simulink library "DC_Loads_Lib"  (R2014a)
settings: Solver=ode45  StartTime=0.0  StopTime=10.0  RelTol=1e-3
undefined symbols (not defined in the file): APN_Param, D1, Delta, Hydride, Metal, Nickel, Ts
libraries: powerlib x30, fl_lib x26, nesl_utility x14, DC_Loads_Lib x3, elec_lib x2, electricdrivelib x1, simulink x1, APN_Battery_Lib x1, sh_lib x1
Description:
  | Copyright 2014 The MathWorks, Inc.
settings Model: Creator=smiller  LastModifiedBy=psanghvi

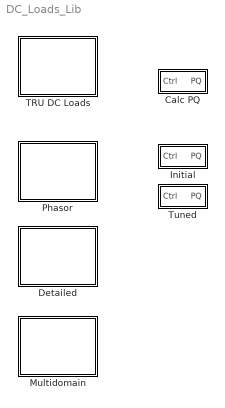
== system DC_Loads_Lib ==
  Calc PQ : Subsystem  BlockChoice=Initial
      settings: TemplateBlock=self  MemberBlocks=Initial,Tuned
  Detailed : Subsystem
      mask Display: image(imread('TRU_Detailed_IMAGE.jpg'));
  Initial : Subsystem
  Multidomain : Subsystem
      mask Display: image(imread('TRU_Multidomain_IMAGE.jpg'));
  Phasor : Subsystem
      mask Display: image(imread('TRU_Phasor_IMAGE.jpg'));
  TRU DC Loads : Subsystem  BlockChoice=Detailed
      settings: TemplateBlock=self  MemberBlocks=Detailed,Multidomain,Phasor
  Tuned : Subsystem

== system DC_Loads_Lib/Calc PQ ==
  Ctrl : Inport
  Initial : DC_Loads_Lib/Initial
  PQ : Outport
  wires:
  Ctrl/1 -> Initial/1
  Initial/1 -> PQ/1

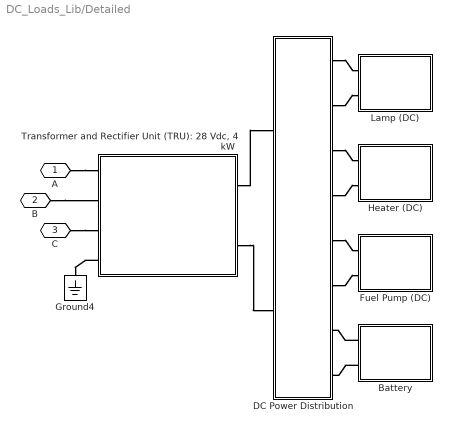
== system DC_Loads_Lib/Detailed ==
  Battery : Subsystem
      mask Display:
      | image(imread('BatteryDC_PS_IMAGE.jpg','jpg'))
      | port_label('LConn',1,'+');
      | port_label('LConn',2,'-');
  "DC Power Distribution " : Subsystem
  Fuel Pump (DC) : Subsystem
      mask Display:
      | image(imread('PumpDC_PS_IMAGE.jpg','jpg'))
      | port_label('LConn',1,'+');
      | port_label('LConn',2,'-');
  Ground4 : powerlib/Elements/Ground  LConnTagsString=a
  Heater (DC) : Subsystem
      mask Display:
      | image(imread('HeaterDC_PS_IMAGE.jpg','jpg'))
      | port_label('LConn',1,'+');
      | port_label('LConn',2,'-');
  Lamp (DC) : Subsystem
      mask Display:
      | image(imread('LampDC_PS_IMAGE.jpg','jpg'))
      | port_label('LConn',1,'+');
      | port_label('LConn',2,'-');
  "Transformer and Rectifier Unit (TRU): 28 Vdc, 4 kW" : Subsystem
      mask Display:
      | image(imread('TRU_PS_IMAGE.jpg','jpg'));
      | port_label('LConn',1,'A');
      | port_label('LConn',2,'B');
      | port_label('LConn',3,'C');
      | port_label('LConn',4,'N');
      | port_label('RConn',1,'+');
      | port_label('RConn',2,'-');
  A : PMIOPort  Port=1  Side=Left
  B : PMIOPort  Port=2  Side=Left
  C : PMIOPort  Port=3  Side=Left
  connections:
  A/RConn1 -- "Transformer and Rectifier Unit (TRU): 28 Vdc, 4 kW"/LConn1
  C/RConn1 -- "Transformer and Rectifier Unit (TRU): 28 Vdc, 4 kW"/LConn3
  B/RConn1 -- "Transformer and Rectifier Unit (TRU): 28 Vdc, 4 kW"/LConn2
  "Transformer and Rectifier Unit (TRU): 28 Vdc, 4 kW"/RConn2 -- "DC Power Distribution "/LConn2
  "DC Power Distribution "/RConn6 -- Fuel Pump (DC)/LConn2
  "DC Power Distribution "/RConn1 -- Lamp (DC)/LConn1
  "DC Power Distribution "/RConn5 -- Fuel Pump (DC)/LConn1
  "DC Power Distribution "/RConn2 -- Lamp (DC)/LConn2
  "Transformer and Rectifier Unit (TRU): 28 Vdc, 4 kW"/RConn1 -- "DC Power Distribution "/LConn1
  "Transformer and Rectifier Unit (TRU): 28 Vdc, 4 kW"/LConn4 -- Ground4/LConn1
  "DC Power Distribution "/RConn3 -- Heater (DC)/LConn1
  "DC Power Distribution "/RConn4 -- Heater (DC)/LConn2
  Battery/LConn1 -- "DC Power Distribution "/RConn7
  Battery/LConn2 -- "DC Power Distribution "/RConn8

== system DC_Loads_Lib/Initial ==
  Ctrl : Inport
  Bus Selector1 : BusSelector  OutputSignals=TRU_B
  Constant : Constant  Value=APN_Param.TRU.P
  Constant1 : Constant  Value=APN_Param.TRU.Q
  Filter : Subsystem  mask(First-order lag supporting vector signals){b=1e-2, x_initial=[APN_Param.TRU.P APN_Param.TRU.Q]*0}
      mask prompts: b "Filter time constant"; x_initial "Initial output"
      mask help: Models a lag of the form 1/(b*s+1) where s is the Laplace operator.
  Mux : Mux  Inputs=2
  Product : Product
  PQ : Outport
  wires:
  Product/1 -> Filter/1(In)
  Filter/1(Out) -> PQ/1
  Bus Selector1/1 -> Product/2  "<TRU_B>"
  Mux/1 -> Product/1
  Ctrl/1 -> Bus Selector1/1
  Constant/1 -> Mux/1
  Constant1/1 -> Mux/2

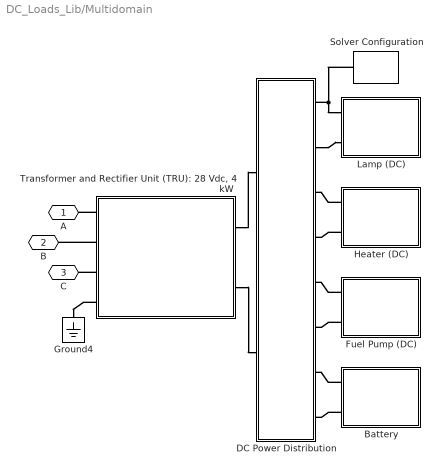
== system DC_Loads_Lib/Multidomain ==
  Battery : Subsystem
      mask Display:
      | image(imread('BatteryDC_SS_IMAGE.jpg','jpg'))
      | port_label('LConn',1,'+');
      | port_label('LConn',2,'-');
  "DC Power Distribution " : Subsystem
  Fuel Pump (DC) : Subsystem
      mask Display:
      | image(imread('PumpDC_SS_IMAGE.jpg','jpg'))
      | port_label('LConn',1,'+');
      | port_label('LConn',2,'-');
  Ground4 : powerlib/Elements/Ground  LConnTagsString=a
  Heater (DC) : Subsystem
      mask Display:
      | image(imread('HeaterDC_SS_IMAGE.jpg','jpg'))
      | port_label('LConn',1,'+');
      | port_label('LConn',2,'-');
  Lamp (DC) : Subsystem
      mask Display:
      | image(imread('LampDC_SS_IMAGE.jpg','jpg'))
      | port_label('LConn',1,'+');
      | port_label('LConn',2,'-');
  Solver Configuration : nesl_utility/Solver Configuration  PhysicalDomain=network_engine_domain  SubClassName=solver  LeftPortType=input  RightPortType=generic  Accelerate=off  Tones=[]  Harmonics=[]  SimulateNoise=off  Profile=off  UseLocalSampling=off  EnableSwitchedLinearOptims=on  FrequencyDomain=off  UseCCode=off  RelTol=0.001  AbsTol=1e-06  MinStep=1e-09  ToWorkspace=off  DoDC=off  ResidualTolerance=1e-9  UseLocalSolver=on  LocalSolverChoice=NE_BACKWARD_EULER_ADVANCER  LocalSolverSampleTime=Ts  DoFixedCost=on  MaxNonlinIter=3  MaxModeIter=2  LinearAlgebra=Sparse  DelaysMemoryBudget=1024  AutomaticFiltering=on  FilteringTimeConstant=0.001
  "Transformer and Rectifier Unit (TRU): 28 Vdc, 4 kW" : Subsystem
      mask Display:
      | image(imread('TRU_PSSS_IMAGE.jpg','jpg'));
      | port_label('LConn',1,'A');
      | port_label('LConn',2,'B');
      | port_label('LConn',3,'C');
      | port_label('LConn',4,'N');
      | port_label('RConn',1,'+');
      | port_label('RConn',2,'-');
  A : PMIOPort  Port=1  Side=Left
  B : PMIOPort  Port=2  Side=Left
  C : PMIOPort  Port=3  Side=Left
  connections:
  Battery/LConn2 -- "DC Power Distribution "/RConn8
  Battery/LConn1 -- "DC Power Distribution "/RConn7
  "Transformer and Rectifier Unit (TRU): 28 Vdc, 4 kW"/RConn2 -- "DC Power Distribution "/LConn2
  "Transformer and Rectifier Unit (TRU): 28 Vdc, 4 kW"/RConn1 -- "DC Power Distribution "/LConn1
  Fuel Pump (DC)/LConn1 -- "DC Power Distribution "/RConn5
  Fuel Pump (DC)/LConn2 -- "DC Power Distribution "/RConn6
  Heater (DC)/LConn1 -- "DC Power Distribution "/RConn3
  Heater (DC)/LConn2 -- "DC Power Distribution "/RConn4
  "DC Power Distribution "/RConn1 -- Lamp (DC)/LConn1 -- Solver Configuration/RConn1
  "DC Power Distribution "/RConn2 -- Lamp (DC)/LConn2
  "Transformer and Rectifier Unit (TRU): 28 Vdc, 4 kW"/LConn1 -- A/RConn1
  "Transformer and Rectifier Unit (TRU): 28 Vdc, 4 kW"/LConn3 -- C/RConn1
  "Transformer and Rectifier Unit (TRU): 28 Vdc, 4 kW"/LConn2 -- B/RConn1
  "Transformer and Rectifier Unit (TRU): 28 Vdc, 4 kW"/LConn4 -- Ground4/LConn1

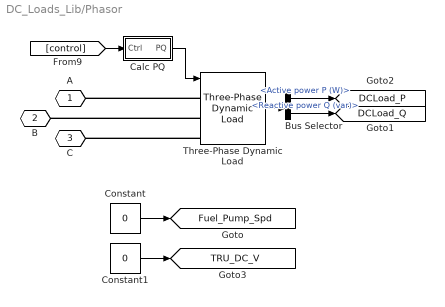
== system DC_Loads_Lib/Phasor ==
  Bus Selector : BusSelector  OutputSignals=Active power P (W),Reactive power Q (var)
  Calc PQ : Subsystem  BlockChoice=Tuned
      settings: AttributesFormatString=%<BlockChoice>  TemplateBlock=DC_Loads_Lib/Calc PQ  MemberBlocks=Initial,Tuned
  Constant : Constant  Value=0
  Constant1 : Constant  Value=0
  Three-Phase Dynamic Load : powerlib/Elements/Three-Phase Dynamic Load  NominalVoltage=[ 500e3 400 ]  ActiveReactivePowers=[APN_Param.TRU.P APN_Param.TRU.Q]  PositiveSequence=[0.0004 0]  ExternalControl=on  NpNq=[1.3 2]  TimeConstants="[0  0  0  0]"  MinimumVoltage=0.7  LoadFlowParameters=[4 0 0 0 0]
  A : PMIOPort  Port=1  Side=Left
  B : PMIOPort  Port=2  Side=Left
  C : PMIOPort  Port=3  Side=Left
  tag scope: DCLoad_P=global, DCLoad_Q=global, Fuel_Pump_Spd=global, TRU_DC_V=global
  wires:
  Bus Selector/1 -> [DCLoad_P]  "<Active power P (W)>"
  Three-Phase Dynamic Load/1 -> Bus Selector/1
  Constant/1 -> [Fuel_Pump_Spd]
  Bus Selector/2 -> [DCLoad_Q]  "<Reactive power Q (var)>"
  [control] -> Calc PQ/1(Ctrl)
  Calc PQ/1(PQ) -> Three-Phase Dynamic Load/1
  Constant1/1 -> [TRU_DC_V]
  connections:
  Three-Phase Dynamic Load/LConn3 -- C/RConn1
  Three-Phase Dynamic Load/LConn2 -- B/RConn1
  Three-Phase Dynamic Load/LConn1 -- A/RConn1

== system DC_Loads_Lib/TRU DC Loads ==
  Detailed : DC_Loads_Lib/Detailed  SystemSampleTime=-1
  A : PMIOPort  Port=1  Side=Left
  B : PMIOPort  Port=2  Side=Left
  C : PMIOPort  Port=3  Side=Left
  connections:
  Detailed/LConn1 -- A/RConn1
  Detailed/LConn2 -- B/RConn1
  Detailed/LConn3 -- C/RConn1

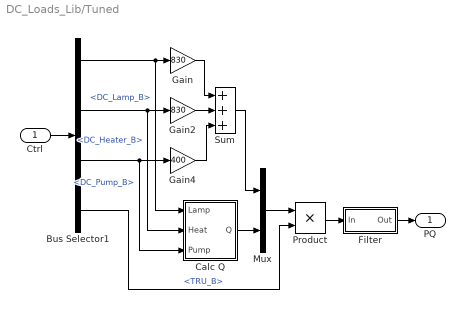
== system DC_Loads_Lib/Tuned ==
  Ctrl : Inport
  Bus Selector1 : BusSelector  OutputSignals=TRU_B_Bus.DC_Lamp_B,TRU_B_Bus.DC_Heater_B,TRU_B_Bus.DC_Pump_B,TRU_B
  Calc Q : Subsystem
  Filter : Subsystem  mask(First-order lag supporting vector signals){b=1e-2, x_initial=0}
      mask prompts: b "Filter time constant"; x_initial "Initial output"
      mask help: Models a lag of the form 1/(b*s+1) where s is the Laplace operator.
  Gain : Gain  Gain=830
  Gain2 : Gain  Gain=830
  Gain4 : Gain  Gain=400
  Mux : Mux  Inputs=2
  Product : Product
  Sum : Sum  Inputs=+++
  PQ : Outport
  wires:
  Ctrl/1 -> Bus Selector1/1
  Bus Selector1/1 -> Calc Q/1(Lamp), Gain/1  "<DC_Lamp_B>"
  Sum/1 -> Mux/1
  Mux/1 -> Product/1
  Bus Selector1/2 -> Calc Q/2(Heat), Gain2/1  "<DC_Heater_B>"
  Bus Selector1/3 -> Calc Q/3(Pump), Gain4/1  "<DC_Pump_B>"
  Gain/1 -> Sum/1
  Gain2/1 -> Sum/2
  Gain4/1 -> Sum/3
  Bus Selector1/4 -> Product/2  "<TRU_B>"
  Filter/1(Out) -> PQ/1
  Product/1 -> Filter/1(In)
  Calc Q/1(Q) -> Mux/2

== system DC_Loads_Lib/Detailed/Battery ==
  Battery : electricdrivelib/Extra Sources/Battery  BatType=Nickel-Metal-Hydride  ShowDetailedParameters=off  NomV=28  NomQ=12  SOC=100  PresetModel=on  MaxQ=12.9231  FullV=32.9831  Dis_rate=2.4  R=0.023333  Normal_OP=11.5385  expZone="[30.3729          2.4]"  Dis_Char=off  current=[1.5 3]  Units=Ampere-hour  Batt_Tr=30
  Terminator : Terminator
  + : PMIOPort  Port=1  Side=Left
  - : PMIOPort  Port=2  Side=Left
  wires:
  Battery/1 -> Terminator/1
  connections:
  Battery/LConn1 -- +/RConn1
  Battery/LConn2 -- -/RConn1

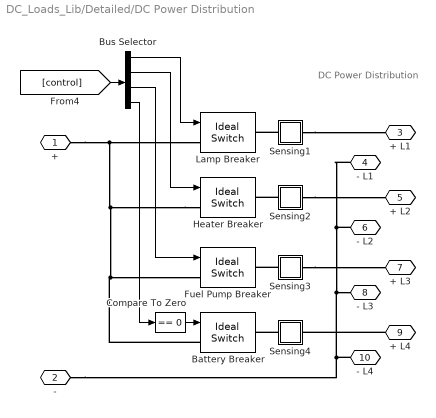
== system DC_Loads_Lib/Detailed/DC Power Distribution  ==
  note: DC Power Distribution
  Battery Breaker : powerlib/Power Electronics/Ideal Switch  Ron=0.001  Lon=0  IC=0  Rs=1e3  Cs=inf  Measurements=off
  Bus Selector : BusSelector  OutputSignals=TRU_B_Bus.DC_Lamp_B,TRU_B_Bus.DC_Heater_B,TRU_B_Bus.DC_Pump_B,TRU_B
  Compare To Zero : simulink/Logic and Bit Operations/Compare To Zero  relop===  OutDataTypeStr=boolean
  Fuel Pump Breaker : powerlib/Power Electronics/Ideal Switch  Ron=0.001  Lon=0  IC=0  Rs=1e3  Cs=inf  Measurements=off
  Heater Breaker : powerlib/Power Electronics/Ideal Switch  Ron=0.001  Lon=0  IC=0  Rs=1e3  Cs=inf  Measurements=off
  Lamp Breaker : powerlib/Power Electronics/Ideal Switch  Ron=0.001  Lon=0  IC=0  Rs=1e3  Cs=inf  Measurements=off
  Sensing1 : Subsystem
      mask Display: disp('S');
  Sensing2 : Subsystem
      mask Display: disp('S');
  Sensing3 : Subsystem
      mask Display: disp('S');
  Sensing4 : Subsystem
      mask Display: disp('S');
  + : PMIOPort  Port=1  Side=Left
  - : PMIOPort  Port=2  Side=Left
  + L1 : PMIOPort  Port=3  Side=Right
  - L1 : PMIOPort  Port=4  Side=Right
  + L2 : PMIOPort  Port=5  Side=Right
  - L2 : PMIOPort  Port=6  Side=Right
  + L3 : PMIOPort  Port=7  Side=Right
  - L3 : PMIOPort  Port=8  Side=Right
  + L4 : PMIOPort  Port=9  Side=Right
  - L4 : PMIOPort  Port=10  Side=Right
  wires:
  Bus Selector/3 -> Fuel Pump Breaker/1
  Bus Selector/2 -> Heater Breaker/1
  Bus Selector/1 -> Lamp Breaker/1
  [control] -> Bus Selector/1
  Bus Selector/4 -> Compare To Zero/1
  Compare To Zero/1 -> Battery Breaker/1
  connections:
  - L2/RConn1 -- - L1/RConn1 -- - L3/RConn1 -- - L4/RConn1 -- -/RConn1
  Heater Breaker/LConn1 -- Battery Breaker/LConn1 -- Fuel Pump Breaker/LConn1 -- Lamp Breaker/LConn1 -- +/RConn1
  Sensing1/LConn1 -- Lamp Breaker/RConn1
  Sensing1/RConn1 -- + L1/RConn1
  Sensing2/LConn1 -- Heater Breaker/RConn1
  Sensing2/RConn1 -- + L2/RConn1
  Sensing3/LConn1 -- Fuel Pump Breaker/RConn1
  Sensing3/RConn1 -- + L3/RConn1
  Sensing4/LConn1 -- Battery Breaker/RConn1
  + L4/RConn1 -- Sensing4/RConn1

== system DC_Loads_Lib/Detailed/Fuel Pump (DC) ==
  Bus Selector : BusSelector  OutputSignals=Speed wm (rad/s)
  DC Machine : powerlib/Machines/DC Machine  PresetModel=No  MechanicalLoad=Torque TL  FieldType=Wound  ShowDetailedParameters=on  MeasurementBus=off  RLa=[ .35 0.0001]  RLf="[ 240  12]"  Laf=1  MachineConstant=Torque constant (N.m/A)  Ke=1.8  Kt=1.8  J=0.0005  Bm=0  Tf=0  w0=0  Ifinit=0  TsPowergui=0  TsBlock=-1
  Gain : Gain  Gain=1.5/200
  + : PMIOPort  Port=1  Side=Left
  - : PMIOPort  Port=2  Side=Left
  tag scope: Fuel_Pump_Spd=global
  wires:
  Bus Selector/1 -> Gain/1, [Fuel_Pump_Spd]  "<Speed wm (rad/s)>"
  DC Machine/1 -> Bus Selector/1
  Gain/1 -> DC Machine/1
  connections:
  DC Machine/LConn2 -- DC Machine/LConn1 -- +/RConn1
  DC Machine/RConn2 -- DC Machine/RConn1 -- -/RConn1

== system DC_Loads_Lib/Detailed/Heater (DC) ==
  note: DC Load
  Series RLC Branch3 : powerlib/Elements/Series RLC Branch  LConnTagsString=__new0  RConnTagsString=__new0  BranchType=R  Resistance=1  Inductance=[]  SetiL0=off  InitialCurrent=0  Capacitance=[]  Setx0=off  InitialVoltage=0  Measurements=Branch voltage and current
  + : PMIOPort  Port=1  Side=Left
  - : PMIOPort  Port=2  Side=Left
  connections:
  +/RConn1 -- Series RLC Branch3/LConn1
  -/RConn1 -- Series RLC Branch3/RConn1

== system DC_Loads_Lib/Detailed/Lamp (DC) ==
  note: DC Load
  Series RLC Branch3 : powerlib/Elements/Series RLC Branch  LConnTagsString=__new0  RConnTagsString=__new0  BranchType=R  Resistance=1  Inductance=[]  SetiL0=off  InitialCurrent=0  Capacitance=[]  Setx0=off  InitialVoltage=0  Measurements=Branch voltage and current
  + : PMIOPort  Port=1  Side=Left
  - : PMIOPort  Port=2  Side=Left
  connections:
  -/RConn1 -- Series RLC Branch3/RConn1
  +/RConn1 -- Series RLC Branch3/LConn1

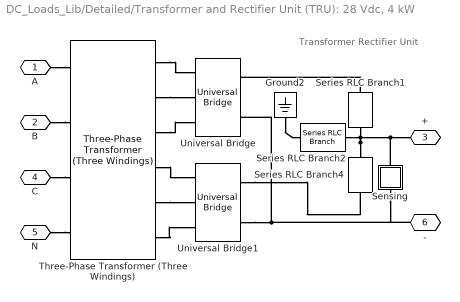
== system DC_Loads_Lib/Detailed/Transformer and Rectifier Unit (TRU): 28 Vdc, 4 kW ==
  note: Transformer Rectifier Unit
  Ground2 : powerlib/Elements/Ground  LConnTagsString=a
  Sensing : Subsystem
  Series RLC Branch1 : powerlib/Elements/Series RLC Branch  LConnTagsString=__new0  RConnTagsString=__new0  BranchType=L  Resistance=[]  Inductance=2e-3  SetiL0=on  InitialCurrent=0  Capacitance=[]  Setx0=off  InitialVoltage=0  Measurements=Branch voltage and current
  Series RLC Branch2 : powerlib/Elements/Series RLC Branch  LConnTagsString=__new0  RConnTagsString=__new0  BranchType=C  Resistance=[]  Inductance=[]  SetiL0=off  InitialCurrent=0  Capacitance=1e-6  Setx0=off  InitialVoltage=0  Measurements=None
  Series RLC Branch4 : powerlib/Elements/Series RLC Branch  LConnTagsString=__new0  RConnTagsString=__new0  BranchType=L  Resistance=[]  Inductance=2e-3  SetiL0=off  InitialCurrent=0  Capacitance=[]  Setx0=off  InitialVoltage=0  Measurements=Branch voltage and current
  Three-Phase Transformer (Three Windings) : powerlib/Elements/Three-Phase Transformer (Three Windings)  Winding1Connection=Yn  UNITS=pu  NominalPower=[ 4200 , 400 ]  Winding1=[ 200 , 0.0002 , 0 ]  Winding2Connection=Delta (D1)  Winding2=[ 22 , 0.0002 , 0 ]  Winding3Connection=Delta (D1)  Winding3=[ 22 , 0.0002 , 0]  SetSaturation=off  Rm=500  Lm=500*10  Saturation=[ 0,0 ; 0.0024,1.2 ; 1.0,1.52 ]  Hysteresis=off  DataFile='hysteresis'  SetInitialFlux=off  InitialFluxes=[0.8 -0.8 0.7]  Measurements=None  MoreParameters=off  BreakLoop=off  DataType=off  TransfoNumber=0
  Universal Bridge : powerlib/Power Electronics/Universal Bridge  Arms=3  SnubberResistance=1e3  SnubberCapacitance=1e-6  Device=Diodes  Ron=1e-3  Lon=0  ForwardVoltages="[  0  0  ]"  ForwardVoltage=0.8  GTOparameters=[ 10e-6 , 20e-6 ]  IGBTparameters=[ 1e-6 , 2e-6 ]  Measurements=None  Measurements_2=None  converterType=Rectifier
  Universal Bridge1 : powerlib/Power Electronics/Universal Bridge  Arms=3  SnubberResistance=1e3  SnubberCapacitance=1e-6  Device=Diodes  Ron=1e-3  Lon=0  ForwardVoltages="[  0  0  ]"  ForwardVoltage=0.8  GTOparameters=[ 10e-6 , 20e-6 ]  IGBTparameters=[ 1e-6 , 2e-6 ]  Measurements=None  Measurements_2=None  converterType=Rectifier
  A : PMIOPort  Port=1  Side=Left
  B : PMIOPort  Port=2  Side=Left
  + : PMIOPort  Port=3  Side=Right
  C : PMIOPort  Port=4  Side=Left
  N : PMIOPort  Port=5  Side=Left
  - : PMIOPort  Port=6  Side=Right
  connections:
  Universal Bridge1/RConn1 -- Series RLC Branch4/RConn1
  Three-Phase Transformer (Three Windings)/RConn6 -- Universal Bridge1/LConn3
  Three-Phase Transformer (Three Windings)/RConn5 -- Universal Bridge1/LConn2
  Three-Phase Transformer (Three Windings)/RConn4 -- Universal Bridge1/LConn1
  Series RLC Branch4/LConn1 -- Sensing/RConn1 -- +/RConn1 -- Series RLC Branch2/LConn1 -- Series RLC Branch1/RConn1
  Series RLC Branch1/LConn1 -- Universal Bridge/RConn1
  N/RConn1 -- Three-Phase Transformer (Three Windings)/LConn4
  C/RConn1 -- Three-Phase Transformer (Three Windings)/LConn3
  B/RConn1 -- Three-Phase Transformer (Three Windings)/LConn2
  A/RConn1 -- Three-Phase Transformer (Three Windings)/LConn1
  Three-Phase Transformer (Three Windings)/RConn3 -- Universal Bridge/LConn3
  Three-Phase Transformer (Three Windings)/RConn2 -- Universal Bridge/LConn2
  Three-Phase Transformer (Three Windings)/RConn1 -- Universal Bridge/LConn1
  Universal Bridge1/RConn2 -- -/RConn1 -- Sensing/LConn1 -- Universal Bridge/RConn2
  Ground2/LConn1 -- Series RLC Branch2/RConn1

== system DC_Loads_Lib/Initial/Filter ==
  In : Inport
  Gain : Gain  Gain=1/b
  Integrator : Integrator  InitialCondition=x_initial
  Sum : Sum  Inputs=|+-  SaturateOnIntegerOverflow=on  InputSameDT=on  OutDataTypeStr=Inherit: Same as first input
  Out : Outport
  wires:
  Gain/1 -> Out/1, Sum/2
  Integrator/1 -> Gain/1
  In/1 -> Sum/1
  Sum/1 -> Integrator/1

== system DC_Loads_Lib/Multidomain/Battery ==
  Ambient temperature : fl_lib/Physical Signals/Sources/PS Constant  constant=273+25
  Battery cell : APN_Battery_Lib/Battery cell  SystemSampleTime=-1
  Convective Heat Transfer : fl_lib/Thermal/Thermal Elements/Convective Heat Transfer  area=Area m^2  heat_tr_coeff=Rtheta W/(m^2 * K)  Q_specify=off  Q_priority=High  Q=0 J/s  T_specify=off  T_priority=High  T=0 K
  Ideal Temperature Source : fl_lib/Thermal/Thermal Sources/Ideal Temperature Source
  Thermal Reference : fl_lib/Thermal/Thermal Elements/Thermal Reference
  + : PMIOPort  Port=1  Side=Left
  - : PMIOPort  Port=2  Side=Left
  connections:
  Battery cell/RConn1 -- -/RConn1
  +/RConn1 -- Battery cell/LConn1
  Thermal Reference/LConn1 -- Ideal Temperature Source/RConn2
  Ideal Temperature Source/RConn1 -- Ambient temperature/RConn1
  Ideal Temperature Source/LConn1 -- Convective Heat Transfer/LConn1
  Convective Heat Transfer/RConn1 -- Battery cell/LConn2

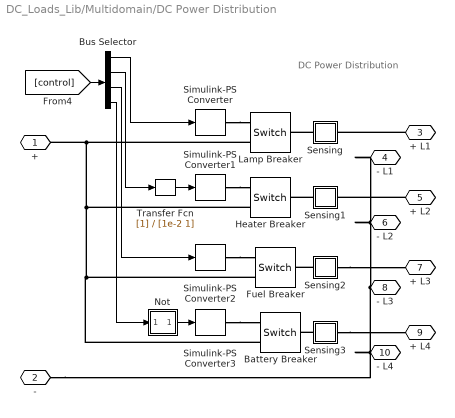
== system DC_Loads_Lib/Multidomain/DC Power Distribution  ==
  note: DC Power Distribution
  Battery Breaker : fl_lib/Electrical/Electrical Elements/Switch  R_closed=0.001 Ohm  G_open=1e-8 1/Ohm  Threshold=0  i_specify=off  i_priority=High  i=0 A  v_specify=off  v_priority=High  v=0 V
  Bus Selector : BusSelector  OutputSignals=TRU_B_Bus.DC_Lamp_B,TRU_B_Bus.DC_Heater_B,TRU_B_Bus.DC_Pump_B,TRU_B
  Fuel Breaker : fl_lib/Electrical/Electrical Elements/Switch  R_closed=0.001 Ohm  G_open=1e-8 1/Ohm  Threshold=0  i_specify=off  i_priority=High  i=0 A  v_specify=off  v_priority=High  v=0 V
  Heater Breaker : fl_lib/Electrical/Electrical Elements/Switch  R_closed=0.001 Ohm  G_open=1e-8 1/Ohm  Threshold=0  i_specify=off  i_priority=High  i=0 A  v_specify=off  v_priority=High  v=0 V
  Lamp Breaker : fl_lib/Electrical/Electrical Elements/Switch  R_closed=0.001 Ohm  G_open=1e-8 1/Ohm  Threshold=0  i_specify=off  i_priority=High  i=0 A  v_specify=off  v_priority=High  v=0 V
  Not : Subsystem
      mask Display: disp('Not')
  Sensing : Subsystem
      mask Display: disp('S');
  Sensing1 : Subsystem
      mask Display: disp('S');
  Sensing2 : Subsystem
      mask Display: disp('S');
  Sensing3 : Subsystem
      mask Display: disp('S');
  Simulink-PS Converter{,1..3} (4 alike) : nesl_utility/Simulink-PS Converter  PhysicalDomain=network_engine_domain  SubClassName=ps_input  LeftPortType=input  RightPortType=output  PseudoPeriodic=off  Frequencies=[]  NoiseDistribution=none  NoiseParameters=[]  Unit=1  AffineConversion=off  InputFiltering=off  SimscapeFilterOrder=1  InputFilterTimeConstant=0.001  UdotUserProvided=1
  Transfer Fcn : TransferFcn  Denominator=[1e-2 1]
  + : PMIOPort  Port=1  Side=Left
  - : PMIOPort  Port=2  Side=Left
  + L1 : PMIOPort  Port=3  Side=Right
  - L1 : PMIOPort  Port=4  Side=Right
  + L2 : PMIOPort  Port=5  Side=Right
  - L2 : PMIOPort  Port=6  Side=Right
  + L3 : PMIOPort  Port=7  Side=Right
  - L3 : PMIOPort  Port=8  Side=Right
  + L4 : PMIOPort  Port=9  Side=Right
  - L4 : PMIOPort  Port=10  Side=Right
  wires:
  Transfer Fcn/1 -> Simulink-PS Converter1/1
  Not/1(Out1) -> Simulink-PS Converter3/1
  Bus Selector/4 -> Not/1(In1)
  [control] -> Bus Selector/1
  Bus Selector/1 -> Simulink-PS Converter/1
  Bus Selector/2 -> Transfer Fcn/1
  Bus Selector/3 -> Simulink-PS Converter2/1
  connections:
  Sensing3/LConn1 -- Battery Breaker/LConn1
  Sensing2/LConn1 -- Fuel Breaker/LConn1
  Simulink-PS Converter3/RConn1 -- Battery Breaker/RConn1
  Simulink-PS Converter2/RConn1 -- Fuel Breaker/RConn1
  Sensing1/LConn1 -- Heater Breaker/LConn1
  Simulink-PS Converter1/RConn1 -- Heater Breaker/RConn1
  + L1/RConn1 -- Sensing/RConn1
  +/RConn1 -- Heater Breaker/RConn2 -- Fuel Breaker/RConn2 -- Battery Breaker/RConn2 -- Lamp Breaker/RConn2
  Sensing/LConn1 -- Lamp Breaker/LConn1
  Simulink-PS Converter/RConn1 -- Lamp Breaker/RConn1
  Sensing3/RConn1 -- + L4/RConn1
  -/RConn1 -- - L4/RConn1 -- - L3/RConn1 -- - L1/RConn1 -- - L2/RConn1
  + L2/RConn1 -- Sensing1/RConn1
  Sensing2/RConn1 -- + L3/RConn1

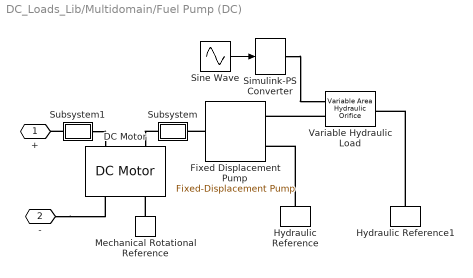
== system DC_Loads_Lib/Multidomain/Fuel Pump (DC) ==
  DC Motor : elec_lib/Actuators & Drivers/Rotational Actuators/DC Motor  parameterization=1  Ra=0.35 Ohm  La=1e-4 H  emf_or_torque=1  Kv=7.2e-5 V/rpm  Ki=6.876e-4 N*m/A  T_stall=2.4e-4 N*m  w_max=1.91e+4 rpm  w_rated=1.5e+4 rpm  P_rated=0.08 W  V_rated=1.5 V  J=5e-4 kg*m^2  lam_param=1  lam=1.5/200 N*m/(rad/s)  i_noload=0 A  V_i_noload=1.5 V  speed0=0 rpm  alpha=0.00393 1/K  Tmeas=25 C  thermal_mass=100 J/K  initial_temperature=25 C
  Fixed Displacement Pump : sh_lib/Pumps and Motors/Fixed-Displacement Pump  D=5e-6 m^3/rad  efficiency_vol=0.92  efficiency_tot=0.8  pr_nominal=1e+7 Pa  w_nominal=188 rad/s  visc_nominal=18 cSt  dens_nominal=900 kg/m^3  k_leak=1e-11 m^3/s/Pa  efficiency_mech=0.7
  Hydraulic Reference : fl_lib/Hydraulic/Hydraulic Elements/Hydraulic Reference
  Hydraulic Reference1 : fl_lib/Hydraulic/Hydraulic Elements/Hydraulic Reference
  Mechanical Rotational Reference : fl_lib/Mechanical/Rotational Elements/Mechanical Rotational Reference
  Simulink-PS Converter : nesl_utility/Simulink-PS Converter  PhysicalDomain=network_engine_domain  SubClassName=ps_input  LeftPortType=input  RightPortType=output  PseudoPeriodic=off  Frequencies=[]  NoiseDistribution=none  NoiseParameters=[]  Unit=1  AffineConversion=off  InputFiltering=on  SimscapeFilterOrder=1  InputFilterTimeConstant=.001  UdotUserProvided=1
  Sine Wave : Sin  Amplitude=1e-4  Bias=1e-3  Frequency=2  SampleTime=0
  Subsystem : Subsystem
      mask Display: disp('S')
  Subsystem1 : Subsystem
      mask Display: disp('S')
  Variable Hydraulic Load : fl_lib/Hydraulic/Hydraulic Elements/Variable Area Hydraulic Orifice  C_d=0.7  Re_cr=12  min_area=1e-12 m^2  q_specify=off  q_priority=High  q=1 m^3/s  p_specify=off  p_priority=High  p=0 Pa
  + : PMIOPort  Port=1  Side=Left
  - : PMIOPort  Port=2  Side=Left
  wires:
  Sine Wave/1 -> Simulink-PS Converter/1
  connections:
  Simulink-PS Converter/RConn1 -- Variable Hydraulic Load/LConn1
  Hydraulic Reference1/LConn1 -- Variable Hydraulic Load/RConn1
  Variable Hydraulic Load/LConn2 -- Fixed Displacement Pump/RConn1
  Hydraulic Reference/LConn1 -- Fixed Displacement Pump/RConn2
  Fixed Displacement Pump/LConn1 -- Subsystem/RConn1
  Subsystem1/RConn1 -- DC Motor/LConn1
  Subsystem1/LConn1 -- +/RConn1
  Subsystem/LConn1 -- DC Motor/LConn2
  Mechanical Rotational Reference/LConn1 -- DC Motor/RConn2
  -/RConn1 -- DC Motor/RConn1

== system DC_Loads_Lib/Multidomain/Heater (DC) ==
  Atmosphere : fl_lib/Thermal/Thermal Elements/Thermal Reference
  Conductive Heat Transfer : fl_lib/Thermal/Thermal Elements/Conductive Heat Transfer  area=1e-4 m^2  thickness=0.1 m  th_cond=401 W/(m*K)  Q_specify=off  Q_priority=High  Q=0 J/s  T_specify=off  T_priority=High  T=0 K
  Convective Heat Transfer : fl_lib/Thermal/Thermal Elements/Convective Heat Transfer  area=1e-4 m^2  heat_tr_coeff=20 W/(m^2 * K)  Q_specify=off  Q_priority=High  Q=0 J/s  T_specify=off  T_priority=High  T=0 K
  Thermal Resistor : elec_lib/Passive Devices/Thermal Resistor  R0=1 Ohm  T0=25 C  alpha=5e-5 1/K  tc=10 s  K_d=0.001 W/K  init_temp=300 K  mc=1 s*W/K
  Thermal Mass : fl_lib/Thermal/Thermal Elements/Thermal Mass  mass=1 kg  sp_heat=447 J/kg/K  Q_specify=off  Q_priority=High  Q=0 J/s  T_specify=on  T_priority=High  T=300 K
  + : PMIOPort  Port=1  Side=Left
  - : PMIOPort  Port=2  Side=Left
  connections:
  Conductive Heat Transfer/LConn1 -- Thermal Resistor/LConn1
  Atmosphere/LConn1 -- Convective Heat Transfer/RConn1
  Conductive Heat Transfer/RConn1 -- Convective Heat Transfer/LConn1 -- Thermal Mass/LConn1
  +/RConn1 -- Thermal Resistor/LConn2
  -/RConn1 -- Thermal Resistor/RConn1

== system DC_Loads_Lib/Multidomain/Lamp (DC) ==
  Simulink-PS Converter : nesl_utility/Simulink-PS Converter  PhysicalDomain=network_engine_domain  SubClassName=ps_input  LeftPortType=input  RightPortType=output  PseudoPeriodic=off  Frequencies=[]  NoiseDistribution=none  NoiseParameters=[]  Unit=1  AffineConversion=off  InputFiltering=on  SimscapeFilterOrder=1  InputFilterTimeConstant=.001  UdotUserProvided=1
  Sine Wave : Sin  Amplitude=0.25  Bias=1  Frequency=2  SampleTime=0
  Variable Resistor : fl_lib/Electrical/Electrical Elements/Variable Resistor  Rmin=0 Ohm  i_specify=off  i_priority=High  i=0 A  v_specify=off  v_priority=High  v=0 V
  + : PMIOPort  Port=1  Side=Left
  - : PMIOPort  Port=2  Side=Left
  wires:
  Sine Wave/1 -> Simulink-PS Converter/1
  connections:
  Simulink-PS Converter/RConn1 -- Variable Resistor/LConn1
  -/RConn1 -- Variable Resistor/RConn1
  +/RConn1 -- Variable Resistor/LConn2

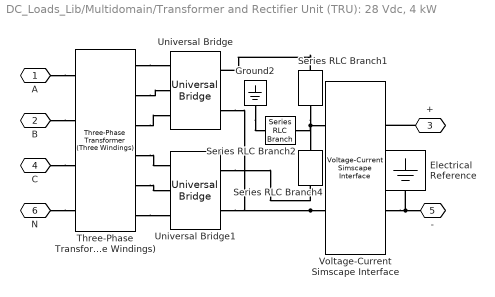
== system DC_Loads_Lib/Multidomain/Transformer and Rectifier Unit (TRU): 28 Vdc, 4 kW ==
  Electrical Reference : fl_lib/Electrical/Electrical Elements/Electrical Reference
  Ground2 : powerlib/Elements/Ground  LConnTagsString=a
  Series RLC Branch1 : powerlib/Elements/Series RLC Branch  LConnTagsString=__new0  RConnTagsString=__new0  BranchType=L  Resistance=[]  Inductance=2e-3  SetiL0=on  InitialCurrent=0  Capacitance=[]  Setx0=off  InitialVoltage=0  Measurements=Branch voltage and current
  Series RLC Branch2 : powerlib/Elements/Series RLC Branch  LConnTagsString=__new0  RConnTagsString=__new0  BranchType=C  Resistance=[]  Inductance=[]  SetiL0=off  InitialCurrent=0  Capacitance=1e-6  Setx0=off  InitialVoltage=0  Measurements=None
  Series RLC Branch4 : powerlib/Elements/Series RLC Branch  LConnTagsString=__new0  RConnTagsString=__new0  BranchType=L  Resistance=[]  Inductance=2e-3  SetiL0=off  InitialCurrent=0  Capacitance=[]  Setx0=off  InitialVoltage=0  Measurements=Branch voltage and current
  Three-Phase Transformer (Three Windings) : powerlib/Elements/Three-Phase Transformer (Three Windings)  Winding1Connection=Yn  UNITS=pu  NominalPower=[ 4200 , 400 ]  Winding1=[ 200 , 0.0002 , 0 ]  Winding2Connection=Delta (D1)  Winding2=[ 22 , 0.0002 , 0 ]  Winding3Connection=Delta (D1)  Winding3=[ 22 , 0.0002 , 0]  SetSaturation=off  Rm=500  Lm=500*10  Saturation=[ 0,0 ; 0.0024,1.2 ; 1.0,1.52 ]  Hysteresis=off  DataFile='hysteresis'  SetInitialFlux=off  InitialFluxes=[0.8 -0.8 0.7]  Measurements=None  MoreParameters=off  BreakLoop=off  DataType=off  TransfoNumber=0
  Universal Bridge : powerlib/Power Electronics/Universal Bridge  Arms=3  SnubberResistance=1e3  SnubberCapacitance=1e-6  Device=Diodes  Ron=1e-3  Lon=0  ForwardVoltages="[  0  0  ]"  ForwardVoltage=0.8  GTOparameters=[ 10e-6 , 20e-6 ]  IGBTparameters=[ 1e-6 , 2e-6 ]  Measurements=None  Measurements_2=None  converterType=Rectifier
  Universal Bridge1 : powerlib/Power Electronics/Universal Bridge  Arms=3  SnubberResistance=1e3  SnubberCapacitance=1e-6  Device=Diodes  Ron=1e-3  Lon=0  ForwardVoltages="[  0  0  ]"  ForwardVoltage=0.8  GTOparameters=[ 10e-6 , 20e-6 ]  IGBTparameters=[ 1e-6 , 2e-6 ]  Measurements=None  Measurements_2=None  converterType=Rectifier
  Voltage-Current Simscape Interface : powerlib/Interface Elements/Voltage-Current Simscape Interface  DFT=off  Fmode=Unit delay (discrete)  T=1e-6  Ts=Ts  i0=0  v0=0  Sd=SimPowerSystems side  Measurements=off
  A : PMIOPort  Port=1  Side=Left
  B : PMIOPort  Port=2  Side=Left
  + : PMIOPort  Port=3  Side=Right
  C : PMIOPort  Port=4  Side=Left
  - : PMIOPort  Port=5  Side=Right
  N : PMIOPort  Port=6  Side=Left
  connections:
  Ground2/LConn1 -- Series RLC Branch2/RConn1
  Voltage-Current Simscape Interface/LConn2 -- Universal Bridge/RConn2 -- Universal Bridge1/RConn2
  Three-Phase Transformer (Three Windings)/RConn1 -- Universal Bridge/LConn1
  Three-Phase Transformer (Three Windings)/RConn2 -- Universal Bridge/LConn2
  Three-Phase Transformer (Three Windings)/RConn3 -- Universal Bridge/LConn3
  A/RConn1 -- Three-Phase Transformer (Three Windings)/LConn1
  B/RConn1 -- Three-Phase Transformer (Three Windings)/LConn2
  C/RConn1 -- Three-Phase Transformer (Three Windings)/LConn3
  Series RLC Branch1/LConn1 -- Universal Bridge/RConn1
  Voltage-Current Simscape Interface/LConn1 -- Series RLC Branch2/LConn1 -- Series RLC Branch4/LConn1 -- Series RLC Branch1/RConn1
  Three-Phase Transformer (Three Windings)/RConn4 -- Universal Bridge1/LConn1
  Three-Phase Transformer (Three Windings)/RConn5 -- Universal Bridge1/LConn2
  Three-Phase Transformer (Three Windings)/RConn6 -- Universal Bridge1/LConn3
  Universal Bridge1/RConn1 -- Series RLC Branch4/RConn1
  +/RConn1 -- Voltage-Current Simscape Interface/RConn1
  -/RConn1 -- Electrical Reference/LConn1 -- Voltage-Current Simscape Interface/RConn2
  N/RConn1 -- Three-Phase Transformer (Three Windings)/LConn4

== system DC_Loads_Lib/Phasor/Calc PQ ==
  Ctrl : Inport
  Tuned : DC_Loads_Lib/Tuned
  PQ : Outport
  wires:
  Ctrl/1 -> Tuned/1
  Tuned/1 -> PQ/1

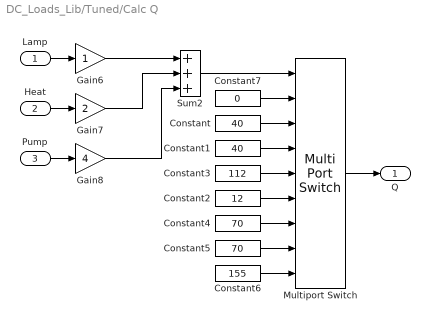
== system DC_Loads_Lib/Tuned/Calc Q ==
  Lamp : Inport
  Heat : Inport  Port=2
  Pump : Inport  Port=3
  Constant : Constant  Value=40
  Constant1 : Constant  Value=40
  Constant2 : Constant  Value=12
  Constant3 : Constant  Value=112
  Constant4 : Constant  Value=70
  Constant5 : Constant  Value=70
  Constant6 : Constant  Value=155
  Constant7 : Constant  Value=0
  Gain6 : Gain
  Gain7 : Gain  Gain=2
  Gain8 : Gain  Gain=4
  Multiport Switch : MultiPortSwitch  DataPortOrder=Zero-based contiguous  Inputs=8
  Sum2 : Sum  Inputs=+++  OutDataTypeStr=int8
  Q : Outport
  wires:
  Gain7/1 -> Sum2/2
  Constant4/1 -> Multiport Switch/7
  Sum2/1 -> Multiport Switch/1
  Constant7/1 -> Multiport Switch/2
  Constant5/1 -> Multiport Switch/8
  Gain8/1 -> Sum2/3
  Constant6/1 -> Multiport Switch/9
  Gain6/1 -> Sum2/1
  Multiport Switch/1 -> Q/1
  Constant3/1 -> Multiport Switch/5
  Constant2/1 -> Multiport Switch/6
  Constant/1 -> Multiport Switch/3
  Constant1/1 -> Multiport Switch/4
  Pump/1 -> Gain8/1
  Lamp/1 -> Gain6/1
  Heat/1 -> Gain7/1

== system DC_Loads_Lib/Tuned/Filter ==
  In : Inport
  Gain : Gain  Gain=1/b
  Integrator : Integrator  InitialCondition=x_initial
  Sum : Sum  Inputs=|+-  SaturateOnIntegerOverflow=on  InputSameDT=on  OutDataTypeStr=Inherit: Same as first input
  Out : Outport
  wires:
  Sum/1 -> Integrator/1
  In/1 -> Sum/1
  Integrator/1 -> Gain/1
  Gain/1 -> Sum/2, Out/1

== system DC_Loads_Lib/Detailed/DC Power Distribution /Sensing1 ==
  Lamp Current Mmt. : powerlib/Measurements/Current Measurement  PhasorSimulation=off  OutputType=Complex  PSBequivalent=0
  + : PMIOPort  Port=1  Side=Left
  - : PMIOPort  Port=2  Side=Right
  tag scope: DC_Lamp_I=global
  wires:
  Lamp Current Mmt./1 -> [DC_Lamp_I]
  connections:
  Lamp Current Mmt./RConn1 -- -/RConn1
  Lamp Current Mmt./LConn1 -- +/RConn1

== system DC_Loads_Lib/Detailed/DC Power Distribution /Sensing2 ==
  Heater Current Mmt. : powerlib/Measurements/Current Measurement  PhasorSimulation=off  OutputType=Complex  PSBequivalent=0
  + : PMIOPort  Port=1  Side=Left
  - : PMIOPort  Port=2  Side=Right
  tag scope: DC_Heater_I=global
  wires:
  Heater Current Mmt./1 -> [DC_Heater_I]
  connections:
  Heater Current Mmt./RConn1 -- -/RConn1
  Heater Current Mmt./LConn1 -- +/RConn1

== system DC_Loads_Lib/Detailed/DC Power Distribution /Sensing3 ==
  Fuel Pump Current Mmt. : powerlib/Measurements/Current Measurement  PhasorSimulation=off  OutputType=Complex  PSBequivalent=0
  + : PMIOPort  Port=1  Side=Left
  - : PMIOPort  Port=2  Side=Right
  tag scope: DC_Pump_I=global
  wires:
  Fuel Pump Current Mmt./1 -> [DC_Pump_I]
  connections:
  Fuel Pump Current Mmt./RConn1 -- -/RConn1
  Fuel Pump Current Mmt./LConn1 -- +/RConn1

== system DC_Loads_Lib/Detailed/DC Power Distribution /Sensing4 ==
  Fuel Pump Current Mmt.1 : powerlib/Measurements/Current Measurement  PhasorSimulation=off  OutputType=Complex  PSBequivalent=0
  + : PMIOPort  Port=1  Side=Left
  - : PMIOPort  Port=2  Side=Right
  tag scope: DC_Battery_I=global
  wires:
  Fuel Pump Current Mmt.1/1 -> [DC_Battery_I]
  connections:
  Fuel Pump Current Mmt.1/LConn1 -- +/RConn1
  -/RConn1 -- Fuel Pump Current Mmt.1/RConn1

== system DC_Loads_Lib/Detailed/Transformer and Rectifier Unit (TRU): 28 Vdc, 4 kW/Sensing ==
  Voltage Measurement : powerlib/Measurements/Voltage Measurement  PhasorSimulation=off  OutputType=Complex  PSBequivalent=0
  + : PMIOPort  Port=1  Side=Right
  - : PMIOPort  Port=2  Side=Left
  tag scope: TRU_DC_V=global
  wires:
  Voltage Measurement/1 -> [TRU_DC_V]
  connections:
  Voltage Measurement/LConn1 -- +/RConn1
  Voltage Measurement/LConn2 -- -/RConn1

== system DC_Loads_Lib/Multidomain/DC Power Distribution /Not ==
  In1 : Inport
  Constant : Constant
  Gain : Gain  Gain=-1
  Sum : Sum  Inputs=|++
  Out1 : Outport
  wires:
  Constant/1 -> Sum/2
  Sum/1 -> Out1/1
  Gain/1 -> Sum/1
  In1/1 -> Gain/1

== system DC_Loads_Lib/Multidomain/DC Power Distribution /Sensing ==
  Current Sensor : fl_lib/Electrical/Electrical Sensors/Current Sensor
  PS-Simulink Converter : nesl_utility/PS-Simulink Converter  PhysicalDomain=network_engine_domain  SubClassName=ps_output  LeftPortType=input  RightPortType=output  PseudoPeriodic=off  Frequencies=[]  Unit=1  AffineConversion=off
  + : PMIOPort  Port=1  Side=Left
  - : PMIOPort  Port=2  Side=Right
  tag scope: DC_Lamp_I=global
  wires:
  PS-Simulink Converter/1 -> [DC_Lamp_I]
  connections:
  Current Sensor/RConn2 -- -/RConn1
  Current Sensor/LConn1 -- +/RConn1
  PS-Simulink Converter/LConn1 -- Current Sensor/RConn1

== system DC_Loads_Lib/Multidomain/DC Power Distribution /Sensing1 ==
  Current Sensor : fl_lib/Electrical/Electrical Sensors/Current Sensor
  PS-Simulink Converter : nesl_utility/PS-Simulink Converter  PhysicalDomain=network_engine_domain  SubClassName=ps_output  LeftPortType=input  RightPortType=output  PseudoPeriodic=off  Frequencies=[]  Unit=1  AffineConversion=off
  + : PMIOPort  Port=1  Side=Left
  - : PMIOPort  Port=2  Side=Right
  tag scope: DC_Heater_I=global
  wires:
  PS-Simulink Converter/1 -> [DC_Heater_I]
  connections:
  PS-Simulink Converter/LConn1 -- Current Sensor/RConn1
  Current Sensor/LConn1 -- +/RConn1
  Current Sensor/RConn2 -- -/RConn1

== system DC_Loads_Lib/Multidomain/DC Power Distribution /Sensing2 ==
  Current Sensor : fl_lib/Electrical/Electrical Sensors/Current Sensor
  PS-Simulink Converter : nesl_utility/PS-Simulink Converter  PhysicalDomain=network_engine_domain  SubClassName=ps_output  LeftPortType=input  RightPortType=output  PseudoPeriodic=off  Frequencies=[]  Unit=1  AffineConversion=off
  + : PMIOPort  Port=1  Side=Left
  - : PMIOPort  Port=2  Side=Right
  tag scope: DC_Pump_I=global
  wires:
  PS-Simulink Converter/1 -> [DC_Pump_I]
  connections:
  Current Sensor/RConn2 -- -/RConn1
  Current Sensor/LConn1 -- +/RConn1
  PS-Simulink Converter/LConn1 -- Current Sensor/RConn1

== system DC_Loads_Lib/Multidomain/DC Power Distribution /Sensing3 ==
  Current Sensor : fl_lib/Electrical/Electrical Sensors/Current Sensor
  PS-Simulink Converter : nesl_utility/PS-Simulink Converter  PhysicalDomain=network_engine_domain  SubClassName=ps_output  LeftPortType=input  RightPortType=output  PseudoPeriodic=off  Frequencies=[]  Unit=1  AffineConversion=off
  + : PMIOPort  Port=1  Side=Left
  - : PMIOPort  Port=2  Side=Right
  tag scope: DC_Battery_I=global
  wires:
  PS-Simulink Converter/1 -> [DC_Battery_I]
  connections:
  PS-Simulink Converter/LConn1 -- Current Sensor/RConn1
  Current Sensor/LConn1 -- +/RConn1
  Current Sensor/RConn2 -- -/RConn1

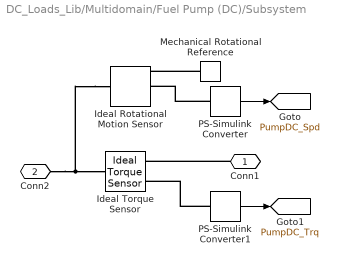
== system DC_Loads_Lib/Multidomain/Fuel Pump (DC)/Subsystem ==
  Ideal Rotational Motion Sensor : fl_lib/Mechanical/Mechanical Sensors/Ideal Rotational Motion Sensor  offset=0 rad
  Ideal Torque Sensor : fl_lib/Mechanical/Mechanical Sensors/Ideal Torque Sensor
  Mechanical Rotational Reference : fl_lib/Mechanical/Rotational Elements/Mechanical Rotational Reference
  PS-Simulink Converter : nesl_utility/PS-Simulink Converter  PhysicalDomain=network_engine_domain  SubClassName=ps_output  LeftPortType=input  RightPortType=output  PseudoPeriodic=off  Frequencies=[]  Unit=1  AffineConversion=off
  PS-Simulink Converter1 : nesl_utility/PS-Simulink Converter  PhysicalDomain=network_engine_domain  SubClassName=ps_output  LeftPortType=input  RightPortType=output  PseudoPeriodic=off  Frequencies=[]  Unit=1  AffineConversion=off
  Conn1 : PMIOPort  Port=1  Side=Right
  Conn2 : PMIOPort  Port=2  Side=Left
  tag scope: PumpDC_Spd=global, PumpDC_Trq=global
  wires:
  PS-Simulink Converter1/1 -> [PumpDC_Trq]
  PS-Simulink Converter/1 -> [PumpDC_Spd]
  connections:
  PS-Simulink Converter/LConn1 -- Ideal Rotational Motion Sensor/RConn2
  Mechanical Rotational Reference/LConn1 -- Ideal Rotational Motion Sensor/RConn1
  PS-Simulink Converter1/LConn1 -- Ideal Torque Sensor/RConn2
  Ideal Rotational Motion Sensor/LConn1 -- Ideal Torque Sensor/LConn1 -- Conn2/RConn1
  Conn1/RConn1 -- Ideal Torque Sensor/RConn1

== system DC_Loads_Lib/Multidomain/Fuel Pump (DC)/Subsystem1 ==
  Current Sensor : fl_lib/Electrical/Electrical Sensors/Current Sensor
  PS-Simulink Converter1 : nesl_utility/PS-Simulink Converter  PhysicalDomain=network_engine_domain  SubClassName=ps_output  LeftPortType=input  RightPortType=output  PseudoPeriodic=off  Frequencies=[]  Unit=1  AffineConversion=off
  Conn1 : PMIOPort  Port=1  Side=Right
  Conn2 : PMIOPort  Port=2  Side=Left
  tag scope: PumpDC_i=global
  wires:
  PS-Simulink Converter1/1 -> [PumpDC_i]
  connections:
  Conn1/RConn1 -- Current Sensor/RConn2
  Conn2/RConn1 -- Current Sensor/LConn1
  PS-Simulink Converter1/LConn1 -- Current Sensor/RConn1
